simulink model "DroneModel"  (R2023a)
settings: Solver=VariableStepAuto  StartTime=0.0  StopTime=10.0  RelTol=1e-3
settings Model: Creator=Henrik  LastModifiedBy=Henrik

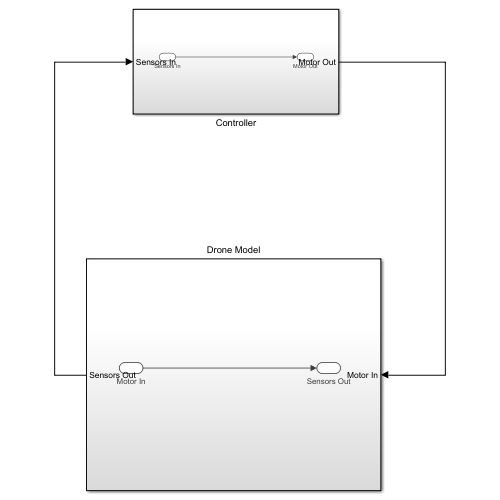
[thumbnail: Simulink's stored preview of the top-level diagram]
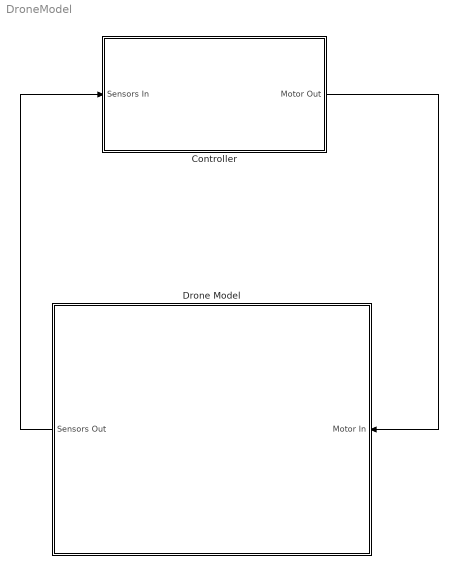
== system DroneModel ==
  Controller : Subsystem
  Drone Model : Subsystem
  wires:
  Controller/1(Motor Out) -> Drone Model/1(Motor In)
  Drone Model/1(Sensors Out) -> Controller/1(Sensors In)

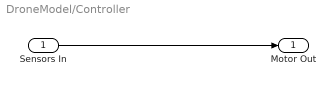
== system DroneModel/Controller ==
  Sensors In : Inport
  Motor Out : Outport
  wires:
  Sensors In/1 -> Motor Out/1

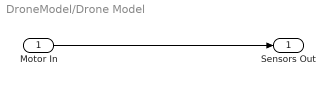
== system DroneModel/Drone Model ==
  Motor In : Inport
  Sensors Out : Outport
  wires:
  Motor In/1 -> Sensors Out/1
